simulink model "srmob_lab_model"  (R2018a)
settings: Solver=ode45  StartTime=0.0  StopTime=2.5  FixedStep=t_pp  MaxStep=0.01  RelTol=1e-3
values from neighbouring files (symbols this model uses):
  inv_J = inv(J)    [srmob_lab_init.m]
  inv_N = inv(N)    [srmob_lab_init.m]
  inv_R_m = inv(R_m)    [srmob_lab_init.m]
  k_c = k_i+50    (= 115.65867657)    [srmob_lab_init.m]
  k_i = (T*omega_0^2) / (K*k_p)    (= 65.6586765699)    [srmob_lab_init.m]
  K_m = [k_m 0; 0 k_m]    [srmob_lab_init.m]
  k_p = 1.0    (= 1)    [VfoControllerPf.m]    (also in VfoControllerPs.m; VfoControllerTt.m; srmob_lab_init.m = 2.52443181818)
  q_initial_conditions = [0; -0.5; -1]    [srmob_lab_init.m]
  T_F = 1/k_i    (= 0.0152302795646)    [srmob_lab_init.m]
  u_initial_conditions = [0; 0]    [srmob_lab_init.m]
  u_max = [u_limit; u_limit]    [srmob_lab_init.m]
  u_min = [-u_limit; -u_limit]    [srmob_lab_init.m]
undefined symbols (not defined in the file or in its folder): Qd01, Qd02, Qd11, Qd12, Qd21, Qd22, Qd31, Qd32
libraries: dsppolyfun x6
settings Model: Creator=szymon  LastModifiedBy=szymon

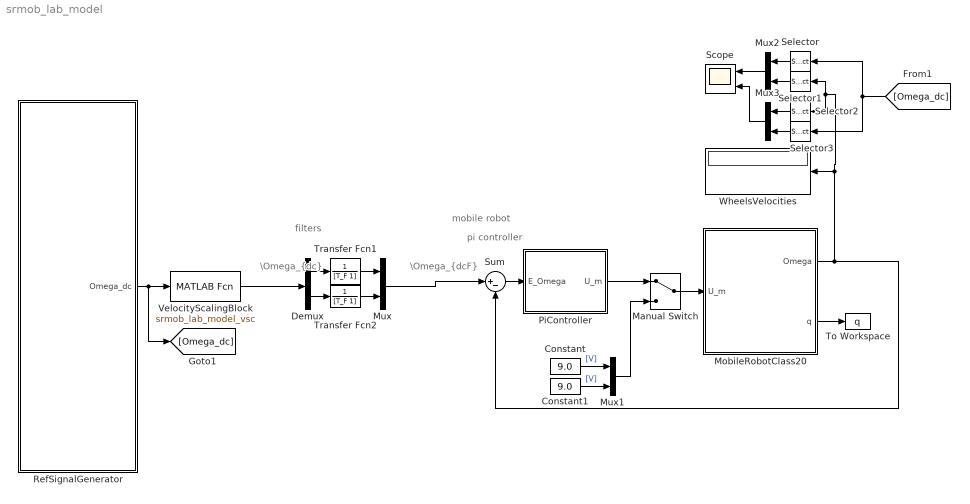
== system srmob_lab_model ==
  note: \Omega_{dc}
  note: \Omega_{dcF}
  note: filters
  note: pi controller
  note: mobile robot
  Constant : Constant  Value=9.0
  Constant1 : Constant  Value=9.0
  Demux : Demux  Outputs=2
  Manual Switch : ManualSwitch
  MobileRobotClass20 : Subsystem
  Mux{,1..3} (4 alike) : Mux  Inputs=2
  PiController : Subsystem
  RefSignalGenerator : Subsystem
  Scope : Scope  NumInputPorts=2
  Selector : Selector  InputPortWidth=2  IndexOptions=Index vector (dialog)  Indices=1  OutputSizes=1
  Selector1 : Selector  InputPortWidth=2  IndexOptions=Index vector (dialog)  Indices=1  OutputSizes=1
  Selector2 : Selector  InputPortWidth=2  IndexOptions=Index vector (dialog)  Indices=2  OutputSizes=1
  Selector3 : Selector  InputPortWidth=2  IndexOptions=Index vector (dialog)  Indices=2  OutputSizes=1
  Sum : Sum  Inputs=|+-
  To Workspace : ToWorkspace  VariableName=q  SampleTime=-1
  Transfer Fcn1 : TransferFcn  Numerator=1  Denominator=[T_F 1]
  Transfer Fcn2 : TransferFcn  Numerator=1  Denominator=[T_F 1]
  VelocityScalingBlock : MATLABFcn  MATLABFcn=srmob_lab_model_vsc
  WheelsVelocities : Display
  wires:
  MobileRobotClass20/1(Omega) -> Selector1/1, Selector2/1, WheelsVelocities/1, Sum/2
  Sum/1 -> PiController/1(E_Omega)
  PiController/1(U_m) -> Manual Switch/1
  Demux/1 -> Transfer Fcn1/1
  Demux/2 -> Transfer Fcn2/1
  Mux/1 -> Sum/1
  Transfer Fcn1/1 -> Mux/1
  Transfer Fcn2/1 -> Mux/2
  RefSignalGenerator/1(Omega_dc) -> [Omega_dc], VelocityScalingBlock/1
  Constant/1 -> Mux1/1  "[V]"
  Constant1/1 -> Mux1/2  "[V]"
  Mux1/1 -> Manual Switch/2
  [Omega_dc] -> Selector3/1, Selector/1
  Selector/1 -> Mux2/1
  Selector1/1 -> Mux2/2
  Selector2/1 -> Mux3/1
  Selector3/1 -> Mux3/2
  Mux2/1 -> Scope/1
  Mux3/1 -> Scope/2
  VelocityScalingBlock/1 -> Demux/1
  Manual Switch/1 -> MobileRobotClass20/1(U_m)
  MobileRobotClass20/2(q) -> To Workspace/1

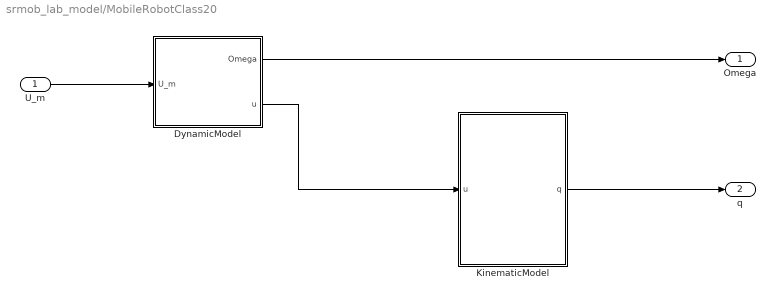
== system srmob_lab_model/MobileRobotClass20 ==
  U_m : Inport
  DynamicModel : Subsystem
  KinematicModel : Subsystem
  Omega : Outport
  q : Outport  Port=2
  wires:
  KinematicModel/1(q) -> q/1
  DynamicModel/2(u) -> KinematicModel/1(u)
  DynamicModel/1(Omega) -> Omega/1
  U_m/1 -> DynamicModel/1(U_m)

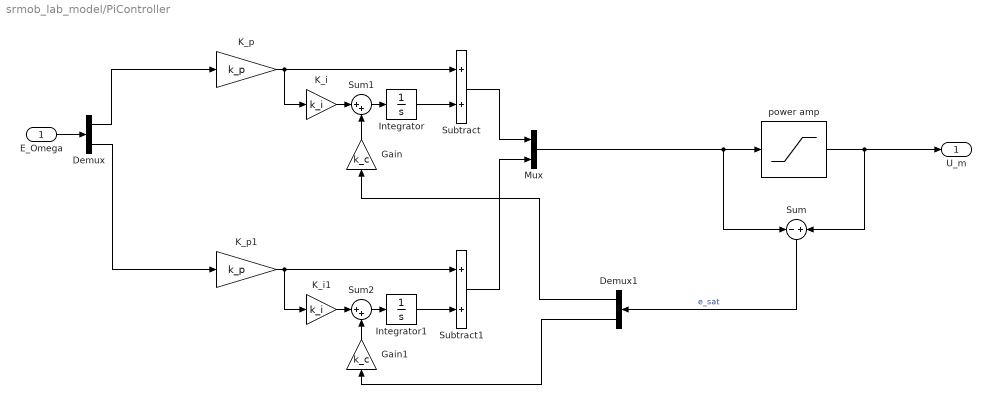
== system srmob_lab_model/PiController ==
  E_Omega : Inport
  Demux : Demux  Outputs=2
  Demux1 : Demux  Outputs=2
  Gain : Gain  Gain=k_c
  Gain1 : Gain  Gain=k_c
  Integrator : Integrator  InitialCondition=[0]
  Integrator1 : Integrator  InitialCondition=[0]
  K_i : Gain  Gain=k_i
  K_i1 : Gain  Gain=k_i
  K_p : Gain  Gain=k_p
  K_p1 : Gain  Gain=k_p
  Mux : Mux  Inputs=2
  Subtract : Sum
  Subtract1 : Sum
  Sum : Sum  Inputs=-+
  Sum1 : Sum  Inputs=|++
  Sum2 : Sum  Inputs=|++
  power amp : Saturate  UpperLimit=u_max  LowerLimit=u_min
  U_m : Outport
  wires:
  Demux/1 -> K_p/1
  Subtract/1 -> Mux/1
  K_i/1 -> Sum1/1
  K_p/1 -> K_i/1, Subtract/1
  Integrator/1 -> Subtract/2
  Demux/2 -> K_p1/1
  Subtract1/1 -> Mux/2
  K_i1/1 -> Sum2/1
  K_p1/1 -> K_i1/1, Subtract1/1
  Integrator1/1 -> Subtract1/2
  Mux/1 -> Sum/1, power amp/1
  E_Omega/1 -> Demux/1
  power amp/1 -> Sum/2, U_m/1
  Sum/1 -> Demux1/1  "e_sat"
  Sum1/1 -> Integrator/1
  Demux1/1 -> Gain/1
  Sum2/1 -> Integrator1/1
  Gain/1 -> Sum1/2
  Gain1/1 -> Sum2/2
  Demux1/2 -> Gain1/1

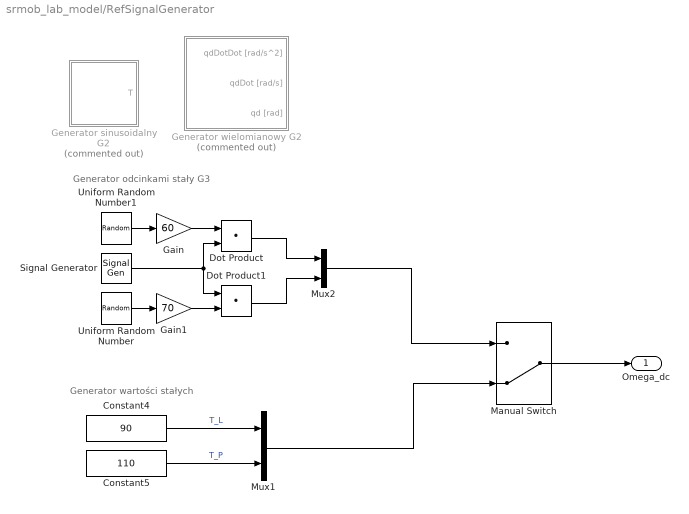
== system srmob_lab_model/RefSignalGenerator ==
  note: Generator
      | wartości stałych
  note: Generator
      | odcinkami stały
      |  G3
  Constant4 : Constant  Value=90
  Constant5 : Constant  Value=110
  Dot Product : DotProduct  InputSameDT=on  OutDataTypeStr=Inherit: Inherit via internal rule
  Dot Product1 : DotProduct  InputSameDT=on  OutDataTypeStr=Inherit: Inherit via internal rule
  Gain : Gain  Gain=60
  Gain1 : Gain  Gain=70
  Generator sinusoidalny G2 : Subsystem  Commented=on
  Generator wielomianowy G2 : Subsystem  Commented=on
  Manual Switch : ManualSwitch  CurrentSetting=0
  Mux1 : Mux  Inputs=2
  Mux2 : Mux  Inputs=2
  Signal Generator : SignalGenerator  WaveForm=square  Units=rad/sec
  Uniform Random Number : UniformRandomNumber  SampleTime=0.5
  Uniform Random Number1 : UniformRandomNumber  SampleTime=0.5
  Omega_dc : Outport
  wires:
  Manual Switch/1 -> Omega_dc/1
  Mux1/1 -> Manual Switch/2
  Mux2/1 -> Manual Switch/1
  Uniform Random Number/1 -> Gain1/1
  Gain/1 -> Dot Product/1
  Uniform Random Number1/1 -> Gain/1
  Dot Product/1 -> Mux2/1
  Gain1/1 -> Dot Product1/2
  Signal Generator/1 -> Dot Product1/1, Dot Product/2
  Dot Product1/1 -> Mux2/2
  Constant5/1 -> Mux1/2  "T_P"
  Constant4/1 -> Mux1/1  "T_L"

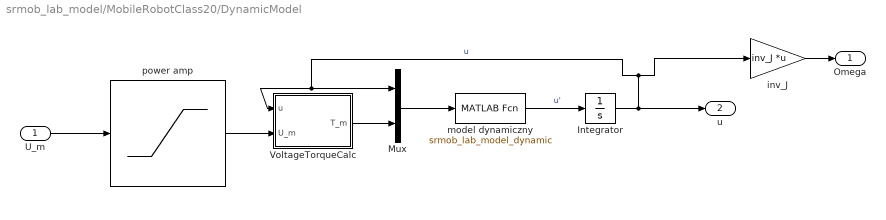
== system srmob_lab_model/MobileRobotClass20/DynamicModel ==
  U_m : Inport
  Integrator : Integrator  InitialCondition=u_initial_conditions
  Mux : Mux  Inputs=2
  VoltageTorqueCalc : Subsystem
  inv_J : Gain  Gain=inv_J  Multiplication=Matrix(K*u) (u vector)
  model dynamiczny : MATLABFcn  MATLABFcn=srmob_lab_model_dynamic
  power amp : Saturate  UpperLimit=u_max  LowerLimit=u_min
  Omega : Outport
  u : Outport  Port=2
  wires:
  Mux/1 -> model dynamiczny/1
  model dynamiczny/1 -> Integrator/1  "u'"
  Integrator/1 -> VoltageTorqueCalc/1(u), Mux/1, inv_J/1, u/1  "u"
  U_m/1 -> power amp/1
  inv_J/1 -> Omega/1
  VoltageTorqueCalc/1(T_m) -> Mux/2
  power amp/1 -> VoltageTorqueCalc/2(U_m)

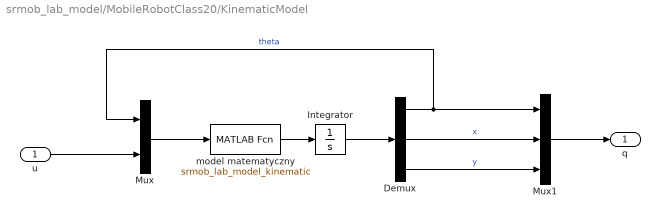
== system srmob_lab_model/MobileRobotClass20/KinematicModel ==
  u : Inport
  Demux : Demux  Outputs=3
  Integrator : Integrator  InitialCondition=q_initial_conditions
  Mux : Mux  Inputs=2
  Mux1 : Mux  Inputs=3
  model matematyczny : MATLABFcn  MATLABFcn=srmob_lab_model_kinematic
  q : Outport
  wires:
  model matematyczny/1 -> Integrator/1
  Mux/1 -> model matematyczny/1
  u/1 -> Mux/2
  Integrator/1 -> Demux/1
  Demux/1 -> Mux/1, Mux1/1  "theta"
  Demux/3 -> Mux1/3  "y"
  Demux/2 -> Mux1/2  "x"
  Mux1/1 -> q/1

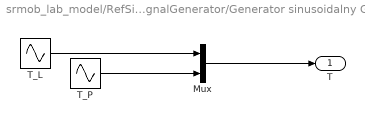
== system srmob_lab_model/RefSignalGenerator/Generator sinusoidalny G2 ==
  Mux : Mux  Inputs=2
  "T_L " : Sin  Frequency=0.5  SampleTime=0
  T_P : Sin  Amplitude=0.5  Frequency=0.25  SampleTime=0
  T : Outport
  wires:
  "T_L "/1 -> Mux/1
  Mux/1 -> T/1
  T_P/1 -> Mux/2

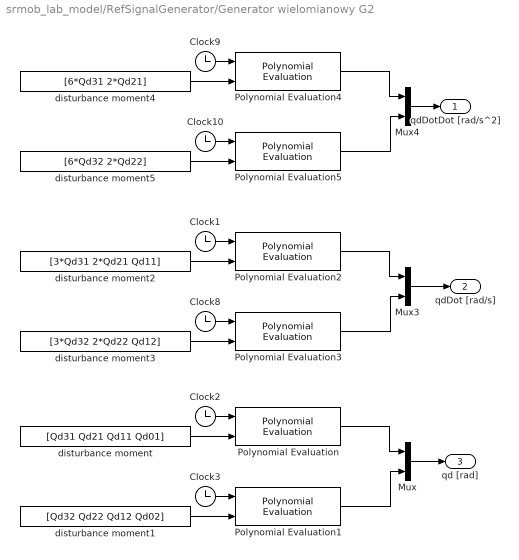
== system srmob_lab_model/RefSignalGenerator/Generator wielomianowy G2 ==
  Clock{1..3,8..10} (6 alike) : Clock
  Mux : Mux  Inputs=2
  Mux3 : Mux  Inputs=2
  Mux4 : Mux  Inputs=2
  Polynomial Evaluation{,1..5} (6 alike) : dsppolyfun/Polynomial Evaluation  useConstCoeffs=off  constCoeffs=[5 4 3 2 1]
      settings: SourceProductName=DSP System Toolbox  SourceProductBaseCode=DS
  disturbance moment : Constant  Value=[Qd31 Qd21 Qd11 Qd01]
  disturbance moment1 : Constant  Value=[Qd32 Qd22 Qd12 Qd02]
  disturbance moment2 : Constant  Value=[3*Qd31 2*Qd21 Qd11]
  disturbance moment3 : Constant  Value=[3*Qd32 2*Qd22 Qd12]
  disturbance moment4 : Constant  Value=[6*Qd31 2*Qd21]
  disturbance moment5 : Constant  Value=[6*Qd32 2*Qd22]
  qdDotDot [rad/s^2] : Outport
  qdDot [rad/s] : Outport  Port=2
  qd [rad] : Outport  Port=3
  wires:
  Mux/1 -> qd [rad]/1
  disturbance moment/1 -> Polynomial Evaluation/2
  disturbance moment1/1 -> Polynomial Evaluation1/2
  Polynomial Evaluation/1 -> Mux/1
  Polynomial Evaluation1/1 -> Mux/2
  Clock2/1 -> Polynomial Evaluation/1
  Clock3/1 -> Polynomial Evaluation1/1
  Mux3/1 -> qdDot [rad/s]/1
  Clock1/1 -> Polynomial Evaluation2/1
  disturbance moment3/1 -> Polynomial Evaluation3/2
  Polynomial Evaluation2/1 -> Mux3/1
  disturbance moment2/1 -> Polynomial Evaluation2/2
  Polynomial Evaluation3/1 -> Mux3/2
  Clock8/1 -> Polynomial Evaluation3/1
  Clock10/1 -> Polynomial Evaluation5/1
  Polynomial Evaluation5/1 -> Mux4/2
  Polynomial Evaluation4/1 -> Mux4/1
  disturbance moment5/1 -> Polynomial Evaluation5/2
  Clock9/1 -> Polynomial Evaluation4/1
  disturbance moment4/1 -> Polynomial Evaluation4/2
  Mux4/1 -> qdDotDot [rad/s^2]/1

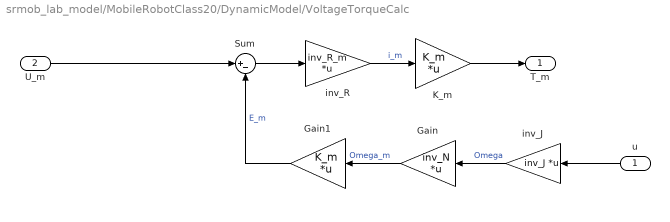
== system srmob_lab_model/MobileRobotClass20/DynamicModel/VoltageTorqueCalc ==
  u : Inport
  U_m : Inport  Port=2
  Gain : Gain  Gain=inv_N  Multiplication=Matrix(K*u) (u vector)
  Gain1 : Gain  Gain=K_m  Multiplication=Matrix(K*u) (u vector)
  K_m : Gain  Gain=K_m  Multiplication=Matrix(K*u) (u vector)
  Sum : Sum  Inputs=|+-
  inv_J : Gain  Gain=inv_J  Multiplication=Matrix(K*u) (u vector)
  inv_R : Gain  Gain=inv_R_m  Multiplication=Matrix(K*u) (u vector)
  T_m : Outport
  wires:
  inv_R/1 -> K_m/1  "i_m"
  Gain/1 -> Gain1/1  "Omega_m"
  inv_J/1 -> Gain/1  "Omega"
  Sum/1 -> inv_R/1
  Gain1/1 -> Sum/2  "E_m"
  K_m/1 -> T_m/1
  u/1 -> inv_J/1
  U_m/1 -> Sum/1
